simulink model "final_26_2_24_Montaldo_simulink"  (R2021a)
settings: Solver=VariableStepAuto  StartTime=0.0  StopTime=10.0  RelTol=1e-3
libraries: cstblocks x1
settings Model: Creator=pedro  LastModifiedBy=pedro

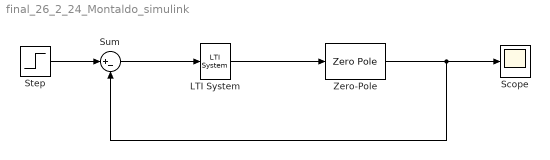
== system final_26_2_24_Montaldo_simulink ==
  LTI System : cstblocks/LTI System  sys=C_d  IC=[]
  Scope : Scope
  Step : Step  SampleTime=0
  Sum : Sum  Inputs=|+-
  Zero-Pole : ZeroPole  Zeros=[]  Poles=[0 0 -80]
  wires:
  Step/1 -> Sum/1
  Sum/1 -> LTI System/1
  LTI System/1 -> Zero-Pole/1
  Zero-Pole/1 -> Sum/2, Scope/1
